simulink model "Model_6"  (R2022b)
settings: Solver=ode4  StartTime=0.0  StopTime=10.0  FixedStep=0.01  RelTol=1e-3
settings Model: Creator=student  LastModifiedBy=Jakub
settings DebuggingCC: UnconnectedInputMsg=warning  UnconnectedOutputMsg=warning  UnconnectedLineMsg=warning
settings ModelReferenceCC: EnableRefExpFcnMdlSchedulingChecks=on
settings RTWCC: DLArmComputeVersion=19.05

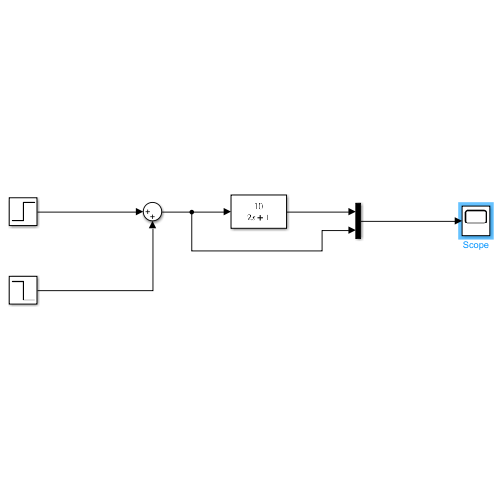
[thumbnail: Simulink's stored preview of the top-level diagram]
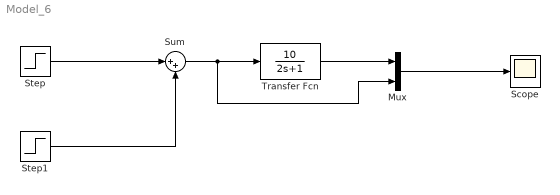
== system Model_6 ==
  Mux : Mux  Inputs=2
  Scope : Scope
  Step : Step  Time=0  After=10  SampleTime=0
  Step1 : Step  Time=0.1  After=-10  SampleTime=0
  Sum : Sum  Inputs=|++
  Transfer Fcn : TransferFcn  Numerator=[10]  Denominator=[2 1]
  wires:
  Mux/1 -> Scope/1
  Transfer Fcn/1 -> Mux/1
  Sum/1 -> Mux/2, Transfer Fcn/1
  Step/1 -> Sum/1
  Step1/1 -> Sum/2
